simulink model "lab02_modelecomplet"  (R2013a)
settings: Solver=ode45  StartTime=0.0  StopTime=3  RelTol=1e-3
values from neighbouring files (symbols this model uses):
  A2 = 20    [Lab02.m]
  kpre = 0.2423076923    [Lab02.m]
  kt = 0.25    [Lab02.m]
settings Model: Creator=ansanf  LastModifiedBy=ToniO
settings DataIOCC: SignalLoggingSaveFormat=ModelDataLogs
settings DebuggingCC: MultiTaskDSMMsg=warning  MultiTaskCondExecSysMsg=none  StateNameClashWarn=none  StrictBusMsg=None
settings RTWCC: IncludeERTFirstTime=on

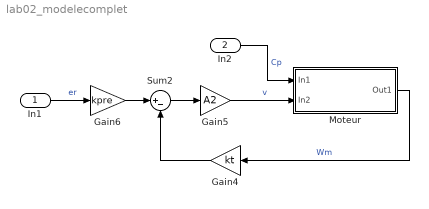
== system lab02_modelecomplet ==
  In1 : Inport
  In2 : Inport  Port=2
  Gain4 : Gain  Gain=kt
  Gain5 : Gain  Gain=A2
  Gain6 : Gain  Gain=kpre
  Moteur : Subsystem
  Sum2 : Sum  Inputs=|+-
  wires:
  Moteur/1(Out1) -> Gain4/1  "Wm"
  Gain6/1 -> Sum2/1
  Sum2/1 -> Gain5/1
  Gain4/1 -> Sum2/2
  Gain5/1 -> Moteur/2(In2)  "v"
  In1/1 -> Gain6/1  "er"
  In2/1 -> Moteur/1(In1)  "Cp"

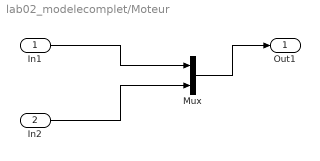
== system lab02_modelecomplet/Moteur ==
  In1 : Inport
  In2 : Inport  Port=2
  Mux : Mux  Inputs=2
  Out1 : Outport
  wires:
  In1/1 -> Mux/1
  In2/1 -> Mux/2
  Mux/1 -> Out1/1
